simulink model "sim_elicottero"  (R2025b)
settings: Solver=VariableStepAuto  StartTime=0.0  StopTime=200  RelTol=1e-3
values from neighbouring files (symbols this model uses):
  A_nom = double(subs(A_sym_nom, [x;u], [x0;u0]))    [dataset_elicottero.m]
  aero = evalin('base','aero')    [analisi_LQG.m]
  alpha_0 = deg2rad(10)    [dataset_elicottero.m]
  B_ext_nom = [B_nom Bd_nom]    [dataset_elicottero.m]
  beta_0 = 0    [dataset_elicottero.m]
  C_angles = [ ... (first row only)    [actuator_lumped_uncertainty.m]    (also in analisi_montecarlo.m = [1 0 0 0; 0 0 1 0]; dataset_elicottero.m)
  Ddec_phys = [8.48868560985e-05  4.80771131122e-11; -3.04359895869e-06  1.06562367592e-06]    [HINF_controllers.mat]    (also in Hinf_hinfstruct.m = Du *      Ddec_scaled *      Du_inv; Hinf_synthesis_full.m = Du *      Ddec_scaled *      inv(Du))
  den_2nd = [1, 2*zeta*omega_n, omega_n^2]    [dataset_elicottero.m]
  denFalpha = [1 24.6158182311]    [HINF_controllers.mat]
  denFbeta = [1 13.1899797029]    [HINF_controllers.mat]
  F1_0 = u0_nom(1)    [dataset_elicottero.m]
  F2_0 = u0_nom(2)    [dataset_elicottero.m]
  HalphaBeta = (C_angle_meas.'*Vinv*C_angle_meas) \      (C_angle_meas.'*Vinv)    [dataset_elicottero.m]
  K_hinfsyn = minreal(          Du *          K_hinfsyn_scaled *          Dy_inv,          1e-7)    [Hinf_hinfstruct.m]    (also in Hinf_synthesis_full.m = minreal(          Du *          K_hinfsyn_scaled *          )
  K_lqg_2dof = ss(      Ac_ctrl,      Bc_ctrl,      Cc_ctrl,      Dc_ctrl)    [LQG_reg_2DOF.m]
  K_lqg_int = ss(      Ac_ctrl,      [Bcr Bcy],      Cc_ctrl,      Dc_ctrl)    [LQG_con_integratore.m]
  K_mix = minreal(          Du *          K_mix_scaled *          Dy_inv,          1e-7)    [Hinf_hinfstruct.m]    (also in Hinf_synthesis_full.m = minreal(          Du *          K_mix_scaled *          Dy_i)
  K_mu = Du * K_mu_scaled * Dy_inv    [mu_synthesis.m]
  Kalpha_tuned = pid(          alphaScaledToPhys *          Kalpha_tuned_scaled.Kp,          alphaScaledToPhys *          Kalpha_tuned_scaled.Ki,          alphaScaledToPhys *          Kalpha_tuned_scaled.Kd,          Kalpha_tuned_scaled.Tf)    [Hinf_hinfstruct.m]    (also in Hinf_synthesis_full.m = pid(          alphaScaledToPhys * Kalpha_tuned_scaled.Kp,   )
  Kbeta_tuned = pid(          betaScaledToPhys *          Kbeta_tuned_scaled.Kp,          betaScaledToPhys *          Kbeta_tuned_scaled.Ki,          betaScaledToPhys *          Kbeta_tuned_scaled.Kd,          Kbeta_tuned_scaled.Tf)    [Hinf_hinfstruct.m]    (also in Hinf_synthesis_full.m = pid(          betaScaledToPhys * Kbeta_tuned_scaled.Kp,     )
  mx_eq = cos(alpha_0) * cos(beta_0)    [dataset_elicottero.m]
  my_eq = -sin(beta_0)    [dataset_elicottero.m]
  num_2nd = omega_n^2    (= 900)    [dataset_elicottero.m]
  numFalpha = [16.7939294955 590.000844903]    [HINF_controllers.mat]
  numFbeta = [34.4835250476 9.60244651319]    [HINF_controllers.mat]
  P_nom_ext = ss(      A_nom,      B_ext_nom,      Cy,      zeros(3,4))    [dataset_elicottero.m]
  tau_d_nom = 0.02    [dataset_elicottero.m]
  umax = 5    [LQG_con_integratore.m]    (also in LQG_reg_1DOF.m; analisi_montecarlo.m = 2.5; dataset_elicottero.m)
  y_acc_eq = -p.g * sin(alpha_0)    [dataset_elicottero.m]
undefined symbols (not defined in the file or in its folder): act, sensor
libraries: simulink x20, slpidlib x2, cstblocks x2
(part 2 of 2)

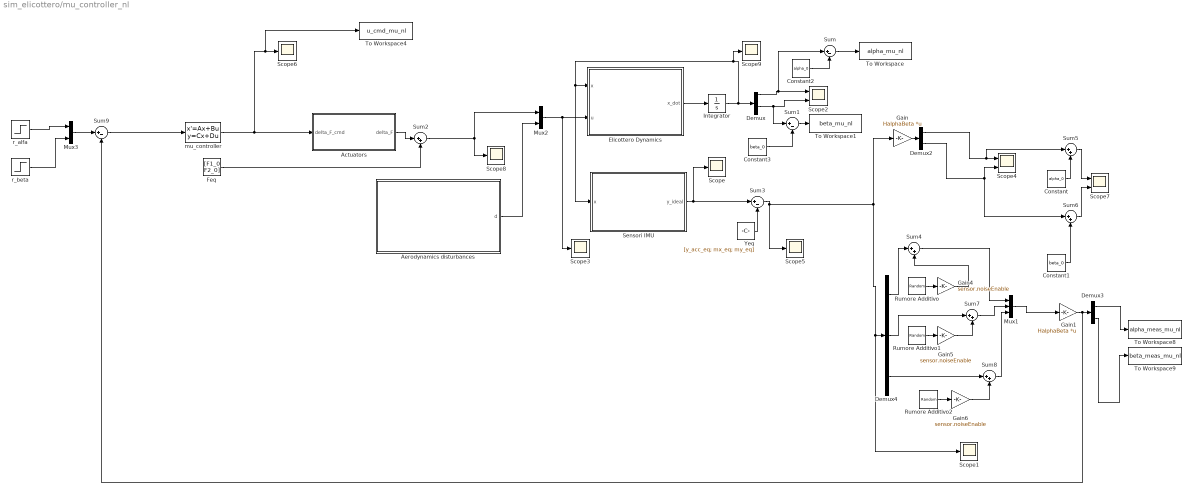
== system sim_elicottero/mu_controller_nl ==
  Actuators : Subsystem
  Aerodynamics disturbances : Subsystem
  Constant : Constant  Value=alpha_0
  Constant1 : Constant  Value=beta_0
  Constant2 : Constant  Value=alpha_0
  Constant3 : Constant  Value=beta_0
  Demux : Demux
  Demux2 : Demux  Outputs=2
  Demux3 : Demux  Outputs=2
  Demux4 : Demux  Outputs=3
  Elicottero Dynamics : MATLAB Function  TreatAsAtomicUnit=on
  Feq : Constant  Value=[F1_0 F2_0]
  Gain : Gain  Gain=HalphaBeta  Multiplication=Matrix(K*u)
  Gain1 : Gain  Gain=HalphaBeta  Multiplication=Matrix(K*u)
  Gain4 : Gain  Gain=sensor.noiseEnable
  Gain5 : Gain  Gain=sensor.noiseEnable
  Gain6 : Gain  Gain=sensor.noiseEnable
  Integrator : Integrator  InitialCondition=[alpha_0; 0; beta_0; 0]
  Mux1 : Mux  Inputs=3
  Mux2 : Mux  Inputs=2
  Mux3 : Mux  Inputs=2
  Rumore Additivo : RandomNumber  Variance=sensor.acc.var  Seed=sensor.seed  SampleTime=sensor.acc.Ts
  Rumore Additivo1 : RandomNumber  Variance=sensor.mag.var  Seed=sensor.seed+1  SampleTime=sensor.mag.Ts
  Rumore Additivo2 : RandomNumber  Variance=sensor.mag.var  Seed=sensor.seed+2  SampleTime=sensor.mag.Ts
  Scope{,1,3,5..6,8..9} (7 alike) : Scope
      Scope settings: ActiveDisplayYMinimum=-2.6695864737629402  ActiveDisplayYMaximum=1.4000873242913907  DataLoggingVariableName=ScopeData14
      Scope1 settings: ActiveDisplayYMinimum=-1.6240661630355766  ActiveDisplayYMaximum=0.25200758348707814  DataLoggingVariableName=ScopeData15
      Scope3 settings: ActiveDisplayYMinimum=-0.066808898460173932  ActiveDisplayYMaximum=0.16260152032849579  DataLoggingVariableName=ScopeData17
      Scope5 settings: ActiveDisplayYMinimum=-0.69850075039123272  ActiveDisplayYMaximum=0.69520204307189137  DataLoggingVariableName=ScopeData20
      Scope6 settings: ActiveDisplayYMinimum=-0.13657354328857155  ActiveDisplayYMaximum=0.3937278655924531  DataLoggingVariableName=ScopeData19
      Scope8 settings: ActiveDisplayYMinimum=-0.16116164249761136  ActiveDisplayYMaximum=0.54820504636646727  DataLoggingVariableName=ScopeData27
      Scope9 settings: ActiveDisplayYMinimum=-0.021816615649929122  ActiveDisplayYMaximum=0.19634954084936207  DataLoggingVariableName=ScopeData28
  Scope2 : Scope  NumInputPorts=2
      settings: ActiveDisplayYMinimum=-0.066338299992033153  ActiveDisplayYMaximum=0.28020406198793696  DataLoggingVariableName=ScopeData16
  Scope4 : Scope  NumInputPorts=2
      settings: ActiveDisplayYMinimum=-0.033068887345671219  ActiveDisplayYMaximum=0.0678695412426075  DataLoggingVariableName=ScopeData18
  Scope7 : Scope  NumInputPorts=2
      settings: ActiveDisplayYMinimum=-0.054885502995600327  ActiveDisplayYMaximum=0.26421908209196954  DataLoggingVariableName=ScopeData26
  Sensori IMU : MATLAB Function  TreatAsAtomicUnit=on
  Sum{,1,3,9} (4 alike) : Sum  Inputs=|+-
  Sum{2,4..8} (6 alike) : Sum  Inputs=|++
  To Workspace : ToWorkspace  VariableName=alpha_mu_nl  SaveFormat=Timeseries  SampleTime=-1
  To Workspace1 : ToWorkspace  VariableName=beta_mu_nl  SaveFormat=Timeseries  SampleTime=-1
  To Workspace4 : ToWorkspace  VariableName=u_cmd_mu_nl  SaveFormat=Timeseries  SampleTime=-1
  To Workspace8 : ToWorkspace  VariableName=alpha_meas_mu_nl  SaveFormat=Timeseries  SampleTime=-1
  To Workspace9 : ToWorkspace  VariableName=beta_meas_mu_nl  SaveFormat=Timeseries  SampleTime=-1
  Yeq : Constant  Value=[y_acc_eq; mx_eq; my_eq]
  mu_controller : StateSpace  A=K_mu.A  B=K_mu.B  C=K_mu.C  D=K_mu.D  InitialCondition=zeros(size(K_mu.A,1),1)
  r_alfa : Step  After=deg2rad(3)  SampleTime=0
  r_beta : Step  After=0  SampleTime=0
  wires:
  mu_controller/1 -> To Workspace4/1, Scope6/1, Actuators/1(delta_F_cmd)
  Mux2/1 -> Scope3/1, Elicottero Dynamics/2(u)
  Aerodynamics disturbances/1(d) -> Mux2/2
  Demux/1 -> Sum/1, Scope2/1
  Demux/3 -> Sum1/1, Scope2/2
  Elicottero Dynamics/1(x_dot) -> Integrator/1
  Integrator/1 -> Scope9/1, Sensori IMU/1(x), Elicottero Dynamics/1(x), Demux/1
  Feq/1 -> Sum2/2
  Sensori IMU/1(y_ideal) -> Sum3/1, Scope/1
  Yeq/1 -> Sum3/2
  Sum7/1 -> Mux1/2
  Constant1/1 -> Sum6/2
  Sum8/1 -> Mux1/3
  Demux4/1 -> Sum4/1
  Rumore Additivo/1 -> Gain4/1
  Gain6/1 -> Sum8/2
  Sum6/1 -> Scope7/2
  Rumore Additivo2/1 -> Gain6/1
  Demux3/2 -> To Workspace9/1
  Rumore Additivo1/1 -> Gain5/1
  Gain5/1 -> Sum7/2
  Demux3/1 -> To Workspace8/1
  Sum4/1 -> Mux1/1
  Demux4/3 -> Sum8/1
  Constant/1 -> Sum5/2
  Demux2/2 -> Sum6/1, Scope4/2
  Demux4/2 -> Sum7/1
  Demux2/1 -> Sum5/1, Scope4/1
  Gain/1 -> Demux2/1
  Sum3/1 -> Demux4/1, Scope1/1, Gain/1, Scope5/1
  Gain4/1 -> Sum4/2
  Sum5/1 -> Scope7/1
  Mux1/1 -> Gain1/1
  Actuators/1(delta_F) -> Sum2/1
  Sum2/1 -> Scope8/1, Mux2/1
  Constant2/1 -> Sum/2
  Sum/1 -> To Workspace/1
  Sum1/1 -> To Workspace1/1
  Constant3/1 -> Sum1/2
  Mux3/1 -> Sum9/1
  r_alfa/1 -> Mux3/1
  r_beta/1 -> Mux3/2
  Sum9/1 -> mu_controller/1
  Gain1/1 -> Sum9/2, Demux3/1

== system sim_elicottero/Hinf_lin/Actuators ==
  delta_F_cmd : Inport
  Band-Limited White Noise : simulink/Sources/Band-Limited White Noise  Cov=act.noisePower_F1  Ts=act.Ts_noise  seed=101
  Band-Limited White Noise1 : simulink/Sources/Band-Limited White Noise  Cov=act.noisePower_F2  Ts=act.Ts_noise  seed=202
  Demux : Demux  Outputs=2
  Gain : Gain  Gain=act.noiseEnable
  Gain1 : Gain  Gain=act.noiseEnable
  Mux : Mux  Inputs=2
  Mux1 : Mux  Inputs=2
  Saturation : Saturate  UpperLimit=act.deltaF1_max  LowerLimit=act.deltaF1_min
  Saturation1 : Saturate  UpperLimit=act.deltaF2_max  LowerLimit=act.deltaF2_min
  Sum1 : Sum  Inputs=|++
  Sum2 : Sum  Inputs=|++
  To Workspace5 : ToWorkspace  VariableName=u_sat_hinf  SaveFormat=Timeseries  SampleTime=-1
  Transfer Fcn : TransferFcn  Numerator=num_2nd  Denominator=den_2nd
  Transfer Fcn1 : TransferFcn  Numerator=num_2nd  Denominator=den_2nd
  Transport Delay1 : TransportDelay  DelayTime=tau_d_nom
  Transport Delay2 : TransportDelay  DelayTime=tau_d_nom
  delta_F : Outport
  wires:
  Gain/1 -> Sum1/2
  Saturation1/1 -> Mux1/2, Transfer Fcn1/1
  Demux/1 -> Saturation/1
  Mux/1 -> delta_F/1
  Transport Delay1/1 -> Sum1/1  "delta_F1"
  Transfer Fcn/1 -> Transport Delay1/1
  Transfer Fcn1/1 -> Transport Delay2/1
  Band-Limited White Noise1/1 -> Gain1/1
  Gain1/1 -> Sum2/2
  Demux/2 -> Saturation1/1
  Transport Delay2/1 -> Sum2/1  "delta_F2"
  delta_F_cmd/1 -> Demux/1
  Band-Limited White Noise/1 -> Gain/1
  Saturation/1 -> Mux1/1, Transfer Fcn/1
  Sum2/1 -> Mux/2
  Sum1/1 -> Mux/1
  Mux1/1 -> To Workspace5/1

== system sim_elicottero/Hinf_lin/Aerodynamics disturbances ==
  Gain : Gain  Gain=aero.enable
  Mux3 : Mux  Inputs=2
  Step : Step  Time=aero.alpha.time  After=aero.alpha.amplitude  SampleTime=0
  Step1 : Step  Time=aero.beta.time  After=aero.beta.amplitude  SampleTime=0
  d : Outport
  wires:
  Step/1 -> Mux3/1
  Mux3/1 -> Gain/1
  Step1/1 -> Mux3/2
  Gain/1 -> d/1

== system sim_elicottero/LQG_1DOF/Actuators ==
  delta_F_cmd : Inport
  Band-Limited White Noise : simulink/Sources/Band-Limited White Noise  Cov=act.noisePower_F1  Ts=act.Ts_noise  seed=101
  Band-Limited White Noise1 : simulink/Sources/Band-Limited White Noise  Cov=act.noisePower_F2  Ts=act.Ts_noise  seed=202
  Demux : Demux  Outputs=2
  Gain : Gain  Gain=act.noiseEnable
  Gain1 : Gain  Gain=act.noiseEnable
  Mux : Mux  Inputs=2
  Mux1 : Mux  Inputs=2
  Saturation : Saturate  UpperLimit=act.deltaF1_max  LowerLimit=act.deltaF1_min
  Saturation1 : Saturate  UpperLimit=act.deltaF2_max  LowerLimit=act.deltaF2_min
  Sum1 : Sum  Inputs=|++
  Sum2 : Sum  Inputs=|++
  To Workspace5 : ToWorkspace  VariableName=u_sat  SaveFormat=Timeseries  SampleTime=-1
  Transfer Fcn : TransferFcn  Numerator=num_2nd  Denominator=den_2nd
  Transfer Fcn1 : TransferFcn  Numerator=num_2nd  Denominator=den_2nd
  Transport Delay1 : TransportDelay  DelayTime=tau_d_nom
  Transport Delay2 : TransportDelay  DelayTime=tau_d_nom
  delta_F : Outport
  wires:
  Gain/1 -> Sum1/2
  Saturation1/1 -> Mux1/2, Transfer Fcn1/1
  Demux/1 -> Saturation/1
  Mux/1 -> delta_F/1
  Transport Delay1/1 -> Sum1/1  "delta_F1"
  Transfer Fcn/1 -> Transport Delay1/1
  Transfer Fcn1/1 -> Transport Delay2/1
  Band-Limited White Noise1/1 -> Gain1/1
  Gain1/1 -> Sum2/2
  Demux/2 -> Saturation1/1
  Transport Delay2/1 -> Sum2/1  "delta_F2"
  delta_F_cmd/1 -> Demux/1
  Band-Limited White Noise/1 -> Gain/1
  Saturation/1 -> Mux1/1, Transfer Fcn/1
  Sum2/1 -> Mux/2
  Sum1/1 -> Mux/1
  Mux1/1 -> To Workspace5/1

== system sim_elicottero/LQG_1DOF/Aerodynamics disturbances ==
  Gain : Gain  Gain=aero.enable
  Mux3 : Mux  Inputs=2
  Step : Step  Time=aero.alpha.time  After=aero.alpha.amplitude  SampleTime=0
  Step1 : Step  Time=aero.beta.time  After=aero.beta.amplitude  SampleTime=0
  d : Outport
  wires:
  Step/1 -> Mux3/1
  Mux3/1 -> Gain/1
  Step1/1 -> Mux3/2
  Gain/1 -> d/1

== system sim_elicottero/LQG_1DOF_nl/Actuators ==
  delta_F_cmd : Inport
  Band-Limited White Noise : simulink/Sources/Band-Limited White Noise  Cov=act.noisePower_F1  Ts=act.Ts_noise  seed=101
  Band-Limited White Noise1 : simulink/Sources/Band-Limited White Noise  Cov=act.noisePower_F2  Ts=act.Ts_noise  seed=202
  Demux : Demux  Outputs=2
  Gain : Gain  Gain=act.noiseEnable
  Gain1 : Gain  Gain=act.noiseEnable
  Mux : Mux  Inputs=2
  Mux1 : Mux  Inputs=2
  Saturation : Saturate  UpperLimit=act.deltaF1_max  LowerLimit=act.deltaF1_min
  Saturation1 : Saturate  UpperLimit=act.deltaF2_max  LowerLimit=act.deltaF2_min
  Sum1 : Sum  Inputs=|++
  Sum2 : Sum  Inputs=|++
  To Workspace5 : ToWorkspace  VariableName=u_sat  SaveFormat=Timeseries  SampleTime=-1
  Transfer Fcn : TransferFcn  Numerator=num_2nd  Denominator=den_2nd
  Transfer Fcn1 : TransferFcn  Numerator=num_2nd  Denominator=den_2nd
  Transport Delay1 : TransportDelay  DelayTime=tau_d_nom
  Transport Delay2 : TransportDelay  DelayTime=tau_d_nom
  delta_F : Outport
  wires:
  Gain/1 -> Sum1/2
  Saturation1/1 -> Mux1/2, Transfer Fcn1/1
  Demux/1 -> Saturation/1
  Mux/1 -> delta_F/1
  Transport Delay1/1 -> Sum1/1  "delta_F1"
  Transfer Fcn/1 -> Transport Delay1/1
  Transfer Fcn1/1 -> Transport Delay2/1
  Band-Limited White Noise1/1 -> Gain1/1
  Gain1/1 -> Sum2/2
  Demux/2 -> Saturation1/1
  Transport Delay2/1 -> Sum2/1  "delta_F2"
  delta_F_cmd/1 -> Demux/1
  Band-Limited White Noise/1 -> Gain/1
  Sum2/1 -> Mux/2
  Sum1/1 -> Mux/1
  Saturation/1 -> Mux1/1, Transfer Fcn/1
  Mux1/1 -> To Workspace5/1

== system sim_elicottero/LQG_1DOF_nl/Aerodynamics disturbances ==
  Gain : Gain  Gain=aero.enable
  Mux3 : Mux  Inputs=2
  Step : Step  Time=aero.alpha.time  After=aero.alpha.amplitude  SampleTime=0
  Step1 : Step  Time=aero.beta.time  After=aero.beta.amplitude  SampleTime=0
  d : Outport
  wires:
  Step/1 -> Mux3/1
  Mux3/1 -> Gain/1
  Step1/1 -> Mux3/2
  Gain/1 -> d/1

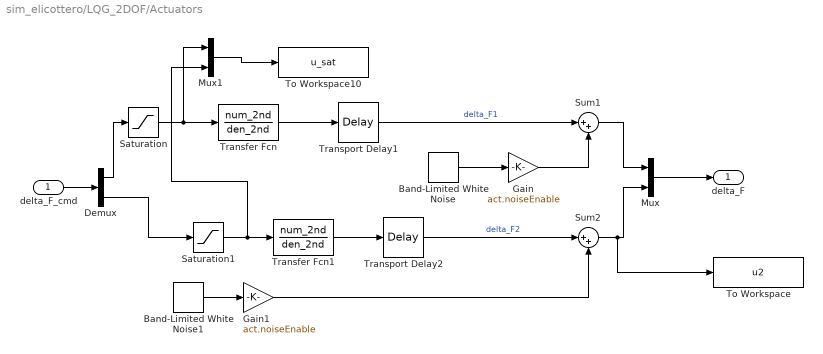
== system sim_elicottero/LQG_2DOF/Actuators ==
  delta_F_cmd : Inport
  Band-Limited White Noise : simulink/Sources/Band-Limited White Noise  Cov=act.noisePower_F1  Ts=act.Ts_noise  seed=101
  Band-Limited White Noise1 : simulink/Sources/Band-Limited White Noise  Cov=act.noisePower_F2  Ts=act.Ts_noise  seed=202
  Demux : Demux  Outputs=2
  Gain : Gain  Gain=act.noiseEnable
  Gain1 : Gain  Gain=act.noiseEnable
  Mux : Mux  Inputs=2
  Mux1 : Mux  Inputs=2
  Saturation : Saturate  UpperLimit=act.deltaF1_max  LowerLimit=act.deltaF1_min
  Saturation1 : Saturate  UpperLimit=act.deltaF2_max  LowerLimit=act.deltaF2_min
  Sum1 : Sum  Inputs=|++
  Sum2 : Sum  Inputs=|++
  To Workspace : ToWorkspace  VariableName=u2  SaveFormat=Timeseries  SampleTime=-1
  To Workspace10 : ToWorkspace  VariableName=u_sat  SaveFormat=Timeseries  SampleTime=-1
  Transfer Fcn : TransferFcn  Numerator=num_2nd  Denominator=den_2nd
  Transfer Fcn1 : TransferFcn  Numerator=num_2nd  Denominator=den_2nd
  Transport Delay1 : TransportDelay  DelayTime=tau_d_nom
  Transport Delay2 : TransportDelay  DelayTime=tau_d_nom
  delta_F : Outport
  wires:
  Gain/1 -> Sum1/2
  Saturation1/1 -> Mux1/2, Transfer Fcn1/1
  Demux/1 -> Saturation/1
  Mux/1 -> delta_F/1
  Transport Delay1/1 -> Sum1/1  "delta_F1"
  Transfer Fcn/1 -> Transport Delay1/1
  Transfer Fcn1/1 -> Transport Delay2/1
  Band-Limited White Noise1/1 -> Gain1/1
  Gain1/1 -> Sum2/2
  Demux/2 -> Saturation1/1
  Transport Delay2/1 -> Sum2/1  "delta_F2"
  delta_F_cmd/1 -> Demux/1
  Band-Limited White Noise/1 -> Gain/1
  Saturation/1 -> Mux1/1, Transfer Fcn/1
  Sum2/1 -> To Workspace/1, Mux/2
  Sum1/1 -> Mux/1
  Mux1/1 -> To Workspace10/1

== system sim_elicottero/LQG_2DOF/Aerodynamics disturbances ==
  Gain : Gain  Gain=aero.enable
  Mux3 : Mux  Inputs=2
  Step : Step  Time=aero.alpha.time  After=aero.alpha.amplitude  SampleTime=0
  Step1 : Step  Time=aero.beta.time  After=aero.beta.amplitude  SampleTime=0
  d : Outport
  wires:
  Step/1 -> Mux3/1
  Mux3/1 -> Gain/1
  Step1/1 -> Mux3/2
  Gain/1 -> d/1

== system sim_elicottero/LQG_2DOF_nl/Actuators ==
  delta_F_cmd : Inport
  Band-Limited White Noise : simulink/Sources/Band-Limited White Noise  Cov=act.noisePower_F1  Ts=act.Ts_noise  seed=101
  Band-Limited White Noise1 : simulink/Sources/Band-Limited White Noise  Cov=act.noisePower_F2  Ts=act.Ts_noise  seed=202
  Demux : Demux  Outputs=2
  Gain : Gain  Gain=act.noiseEnable
  Gain1 : Gain  Gain=act.noiseEnable
  Mux : Mux  Inputs=2
  Saturation : Saturate  UpperLimit=act.deltaF1_max  LowerLimit=act.deltaF1_min
  Saturation1 : Saturate  UpperLimit=act.deltaF2_max  LowerLimit=act.deltaF2_min
  Sum1 : Sum  Inputs=|++
  Sum2 : Sum  Inputs=|++
  To Workspace : ToWorkspace  VariableName=u2  SaveFormat=Timeseries  SampleTime=-1
  Transfer Fcn : TransferFcn  Numerator=num_2nd  Denominator=den_2nd
  Transfer Fcn1 : TransferFcn  Numerator=num_2nd  Denominator=den_2nd
  Transport Delay1 : TransportDelay  DelayTime=tau_d_nom
  Transport Delay2 : TransportDelay  DelayTime=tau_d_nom
  delta_F : Outport
  wires:
  Gain/1 -> Sum1/2
  Saturation1/1 -> Transfer Fcn1/1
  Demux/1 -> Saturation/1
  Mux/1 -> delta_F/1
  Transport Delay1/1 -> Sum1/1  "delta_F1"
  Transfer Fcn/1 -> Transport Delay1/1
  Transfer Fcn1/1 -> Transport Delay2/1
  Band-Limited White Noise1/1 -> Gain1/1
  Gain1/1 -> Sum2/2
  Demux/2 -> Saturation1/1
  Transport Delay2/1 -> Sum2/1  "delta_F2"
  delta_F_cmd/1 -> Demux/1
  Band-Limited White Noise/1 -> Gain/1
  Saturation/1 -> Transfer Fcn/1
  Sum2/1 -> To Workspace/1, Mux/2
  Sum1/1 -> Mux/1

== system sim_elicottero/LQG_2DOF_nl/Aerodynamics disturbances ==
  Gain : Gain  Gain=aero.enable
  Mux3 : Mux  Inputs=2
  Step : Step  Time=aero.alpha.time  After=aero.alpha.amplitude  SampleTime=0
  Step1 : Step  Time=aero.beta.time  After=aero.beta.amplitude  SampleTime=0
  d : Outport
  wires:
  Step/1 -> Mux3/1
  Mux3/1 -> Gain/1
  Step1/1 -> Mux3/2
  Gain/1 -> d/1

== system sim_elicottero/LQG_int/Actuators ==
  delta_F_cmd : Inport
  Band-Limited White Noise : simulink/Sources/Band-Limited White Noise  Cov=act.noisePower_F1  Ts=act.Ts_noise  seed=101
  Band-Limited White Noise1 : simulink/Sources/Band-Limited White Noise  Cov=act.noisePower_F2  Ts=act.Ts_noise  seed=202
  Demux : Demux  Outputs=2
  Gain : Gain  Gain=act.noiseEnable
  Gain1 : Gain  Gain=act.noiseEnable
  Mux : Mux  Inputs=2
  Mux1 : Mux  Inputs=2
  Saturation : Saturate  UpperLimit=act.deltaF1_max  LowerLimit=act.deltaF1_min
  Saturation1 : Saturate  UpperLimit=act.deltaF2_max  LowerLimit=act.deltaF2_min
  Sum1 : Sum  Inputs=|++
  Sum2 : Sum  Inputs=|++
  To Workspace5 : ToWorkspace  VariableName=u_sat  SaveFormat=Timeseries  SampleTime=-1
  Transfer Fcn : TransferFcn  Numerator=num_2nd  Denominator=den_2nd
  Transfer Fcn1 : TransferFcn  Numerator=num_2nd  Denominator=den_2nd
  Transport Delay1 : TransportDelay  DelayTime=tau_d_nom
  Transport Delay2 : TransportDelay  DelayTime=tau_d_nom
  delta_F : Outport
  wires:
  Gain/1 -> Sum1/2
  Saturation1/1 -> Mux1/2, Transfer Fcn1/1
  Demux/1 -> Saturation/1
  Mux/1 -> delta_F/1
  Transport Delay1/1 -> Sum1/1  "delta_F1"
  Transfer Fcn/1 -> Transport Delay1/1
  Transfer Fcn1/1 -> Transport Delay2/1
  Band-Limited White Noise1/1 -> Gain1/1
  Gain1/1 -> Sum2/2
  Demux/2 -> Saturation1/1
  Transport Delay2/1 -> Sum2/1  "delta_F2"
  delta_F_cmd/1 -> Demux/1
  Band-Limited White Noise/1 -> Gain/1
  Saturation/1 -> Mux1/1, Transfer Fcn/1
  Sum2/1 -> Mux/2
  Sum1/1 -> Mux/1
  Mux1/1 -> To Workspace5/1

== system sim_elicottero/LQG_int/Aerodynamics disturbances ==
  Gain : Gain  Gain=aero.enable
  Mux3 : Mux  Inputs=2
  Step : Step  Time=aero.alpha.time  After=aero.alpha.amplitude  SampleTime=0
  Step1 : Step  Time=aero.beta.time  After=aero.beta.amplitude  SampleTime=0
  d : Outport
  wires:
  Step/1 -> Mux3/1
  Mux3/1 -> Gain/1
  Step1/1 -> Mux3/2
  Gain/1 -> d/1

== system sim_elicottero/LQG_int_nl/Actuators ==
  delta_F_cmd : Inport
  Band-Limited White Noise : simulink/Sources/Band-Limited White Noise  Cov=act.noisePower_F1  Ts=act.Ts_noise  seed=101
  Band-Limited White Noise1 : simulink/Sources/Band-Limited White Noise  Cov=act.noisePower_F2  Ts=act.Ts_noise  seed=202
  Demux : Demux  Outputs=2
  Gain : Gain  Gain=act.noiseEnable
  Gain1 : Gain  Gain=act.noiseEnable
  Mux : Mux  Inputs=2
  Mux1 : Mux  Inputs=2
  Saturation : Saturate  UpperLimit=act.deltaF1_max  LowerLimit=act.deltaF1_min
  Saturation1 : Saturate  UpperLimit=act.deltaF2_max  LowerLimit=act.deltaF2_min
  Sum1 : Sum  Inputs=|++
  Sum2 : Sum  Inputs=|++
  To Workspace5 : ToWorkspace  VariableName=u_sat_nl  SaveFormat=Timeseries  SampleTime=-1
  Transfer Fcn : TransferFcn  Numerator=num_2nd  Denominator=den_2nd
  Transfer Fcn1 : TransferFcn  Numerator=num_2nd  Denominator=den_2nd
  Transport Delay1 : TransportDelay  DelayTime=tau_d_nom
  Transport Delay2 : TransportDelay  DelayTime=tau_d_nom
  delta_F : Outport
  wires:
  Gain/1 -> Sum1/2
  Saturation1/1 -> Mux1/2, Transfer Fcn1/1
  Demux/1 -> Saturation/1
  Mux/1 -> delta_F/1
  Transport Delay1/1 -> Sum1/1  "delta_F1"
  Transfer Fcn/1 -> Transport Delay1/1
  Transfer Fcn1/1 -> Transport Delay2/1
  Band-Limited White Noise1/1 -> Gain1/1
  Gain1/1 -> Sum2/2
  Demux/2 -> Saturation1/1
  Transport Delay2/1 -> Sum2/1  "delta_F2"
  delta_F_cmd/1 -> Demux/1
  Band-Limited White Noise/1 -> Gain/1
  Sum2/1 -> Mux/2
  Sum1/1 -> Mux/1
  Saturation/1 -> Mux1/1, Transfer Fcn/1
  Mux1/1 -> To Workspace5/1

== system sim_elicottero/LQG_int_nl/Aerodynamics disturbances ==
  Gain : Gain  Gain=aero.enable
  Mux3 : Mux  Inputs=2
  Step : Step  Time=aero.alpha.time  After=aero.alpha.amplitude  SampleTime=0
  Step1 : Step  Time=aero.beta.time  After=aero.beta.amplitude  SampleTime=0
  d : Outport
  wires:
  Step/1 -> Mux3/1
  Mux3/1 -> Gain/1
  Step1/1 -> Mux3/2
  Gain/1 -> d/1

== system sim_elicottero/mu_controller/Actuators ==
  delta_F_cmd : Inport
  Band-Limited White Noise : simulink/Sources/Band-Limited White Noise  Cov=act.noisePower_F1  Ts=act.Ts_noise  seed=101
  Band-Limited White Noise1 : simulink/Sources/Band-Limited White Noise  Cov=act.noisePower_F2  Ts=act.Ts_noise  seed=202
  Demux : Demux  Outputs=2
  Gain : Gain  Gain=act.noiseEnable
  Gain1 : Gain  Gain=act.noiseEnable
  Mux : Mux  Inputs=2
  Mux1 : Mux  Inputs=2
  Saturation : Saturate  UpperLimit=act.deltaF1_max  LowerLimit=act.deltaF1_min
  Saturation1 : Saturate  UpperLimit=act.deltaF2_max  LowerLimit=act.deltaF2_min
  Sum1 : Sum  Inputs=|++
  Sum2 : Sum  Inputs=|++
  To Workspace5 : ToWorkspace  VariableName=u_sat  SaveFormat=Timeseries  SampleTime=-1
  Transfer Fcn : TransferFcn  Numerator=num_2nd  Denominator=den_2nd
  Transfer Fcn1 : TransferFcn  Numerator=num_2nd  Denominator=den_2nd
  Transport Delay1 : TransportDelay  DelayTime=tau_d_nom
  Transport Delay2 : TransportDelay  DelayTime=tau_d_nom
  delta_F : Outport
  wires:
  Gain/1 -> Sum1/2
  Saturation1/1 -> Mux1/2, Transfer Fcn1/1
  Demux/1 -> Saturation/1
  Mux/1 -> delta_F/1
  Transport Delay1/1 -> Sum1/1  "delta_F1"
  Transfer Fcn/1 -> Transport Delay1/1
  Transfer Fcn1/1 -> Transport Delay2/1
  Band-Limited White Noise1/1 -> Gain1/1
  Gain1/1 -> Sum2/2
  Demux/2 -> Saturation1/1
  Transport Delay2/1 -> Sum2/1  "delta_F2"
  delta_F_cmd/1 -> Demux/1
  Band-Limited White Noise/1 -> Gain/1
  Saturation/1 -> Mux1/1, Transfer Fcn/1
  Sum2/1 -> Mux/2
  Sum1/1 -> Mux/1
  Mux1/1 -> To Workspace5/1

== system sim_elicottero/mu_controller/Aerodynamics disturbances ==
  Gain : Gain  Gain=aero.enable
  Mux3 : Mux  Inputs=2
  Step : Step  Time=aero.alpha.time  After=aero.alpha.amplitude  SampleTime=0
  Step1 : Step  Time=aero.beta.time  After=aero.beta.amplitude  SampleTime=0
  d : Outport
  wires:
  Step/1 -> Mux3/1
  Mux3/1 -> Gain/1
  Step1/1 -> Mux3/2
  Gain/1 -> d/1

== system sim_elicottero/mu_controller_nl/Actuators ==
  delta_F_cmd : Inport
  Band-Limited White Noise : simulink/Sources/Band-Limited White Noise  Cov=act.noisePower_F1  Ts=act.Ts_noise  seed=101
  Band-Limited White Noise1 : simulink/Sources/Band-Limited White Noise  Cov=act.noisePower_F2  Ts=act.Ts_noise  seed=202
  Demux : Demux  Outputs=2
  Gain : Gain  Gain=act.noiseEnable
  Gain1 : Gain  Gain=act.noiseEnable
  Mux : Mux  Inputs=2
  Mux1 : Mux  Inputs=2
  Saturation : Saturate  UpperLimit=act.deltaF1_max  LowerLimit=act.deltaF1_min
  Saturation1 : Saturate  UpperLimit=act.deltaF2_max  LowerLimit=act.deltaF2_min
  Sum1 : Sum  Inputs=|++
  Sum2 : Sum  Inputs=|++
  To Workspace5 : ToWorkspace  VariableName=u_sat_nl  SaveFormat=Timeseries  SampleTime=-1
  Transfer Fcn : TransferFcn  Numerator=num_2nd  Denominator=den_2nd
  Transfer Fcn1 : TransferFcn  Numerator=num_2nd  Denominator=den_2nd
  Transport Delay1 : TransportDelay  DelayTime=tau_d_nom
  Transport Delay2 : TransportDelay  DelayTime=tau_d_nom
  delta_F : Outport
  wires:
  Gain/1 -> Sum1/2
  Saturation1/1 -> Mux1/2, Transfer Fcn1/1
  Demux/1 -> Saturation/1
  Mux/1 -> delta_F/1
  Transport Delay1/1 -> Sum1/1  "delta_F1"
  Transfer Fcn/1 -> Transport Delay1/1
  Transfer Fcn1/1 -> Transport Delay2/1
  Band-Limited White Noise1/1 -> Gain1/1
  Gain1/1 -> Sum2/2
  Demux/2 -> Saturation1/1
  Transport Delay2/1 -> Sum2/1  "delta_F2"
  delta_F_cmd/1 -> Demux/1
  Band-Limited White Noise/1 -> Gain/1
  Sum2/1 -> Mux/2
  Sum1/1 -> Mux/1
  Saturation/1 -> Mux1/1, Transfer Fcn/1
  Mux1/1 -> To Workspace5/1

== system sim_elicottero/mu_controller_nl/Aerodynamics disturbances ==
  Gain : Gain  Gain=aero.enable
  Mux3 : Mux  Inputs=2
  Step : Step  Time=aero.alpha.time  After=aero.alpha.amplitude  SampleTime=0
  Step1 : Step  Time=aero.beta.time  After=aero.beta.amplitude  SampleTime=0
  d : Outport
  wires:
  Step/1 -> Mux3/1
  Mux3/1 -> Gain/1
  Step1/1 -> Mux3/2
  Gain/1 -> d/1

== matlab function sim_elicottero/Hinf_nl/Sensori IMU ==
  data: x input; y_ideal output; p parameter
function y_ideal = sensori_imu(x, p)
    % ESTRAZIONE STATI RILEVANTI
    alpha = x(1);
    beta = x(3);
    
    % EQUAZIONI DEI SENSORI (Misure ideali a 3 uscite)
    y_acc = -p.g * sin(alpha);
    mx = cos(alpha) * cos(beta);
    my = -sin(beta);
    
    % USCITA: Vettore colonna 3x1
    y_ideal = [y_acc; mx; my];
end

== matlab function sim_elicottero/mu_controller_nl/Elicottero Dynamics ==
  data: x input; u input; x_dot output; p parameter
function x_dot = elicottero_dynamics(x, u, p)
    % ESTRAZIONE STATI
    alpha = x(1);
    alpha_dot = x(2);
    beta = x(3);
    beta_dot = x(4);
    
    % ESTRAZIONE INGRESSI

    F1 = u(1);
    F2 = u(2);

    d_alpha = u(3);
    d_beta  = u(4);
                 
    % 1. Vettore velocità angolare nel sistema Body (omega_B)
    % Il Pitch (alpha_dot) ruota attorno all'asse Y_body.
    % Lo Yaw (beta_dot) ruota attorno all'asse Z_inerziale, che proiettato in Body diventa [-sin(alpha); 0; cos(alpha)]
    omega_body = [-beta_dot * sin(alpha); 
                   alpha_dot; 
                   beta_dot * cos(alpha)];
                   
    % 2. Vettore posizione del centro aerodinamico (i rotori a distanza l sull'asse X_body)
    r_cp = [p.l; 0; 0];
    
    % 3. Velocità lineare del corpo dovuta alla rotazione (v = omega x r)
    v_corpo_body = cross(omega_body, r_cp); 
    % (Il risultato analitico sarà: [0; p.l * beta_dot * cos(alpha); -p.l * alpha_dot])
    
    
    % 5. VELOCITÀ RELATIVA VERA (Vento esterno - Velocità del corpo)
    v_rel_body  = - v_corpo_body; 
    v_rel_norm  = norm(v_rel_body);
    
    % Calcolo Forze Aerodinamiche
    % NOTA: Per pulizia del codice, in futuro potresti spostare rho e Cd_A 
    % all'interno della struct dei parametri 'p'
    rho = 1.225; % Densità dell'aria [kg/m^3]
    Cd_A = [0.5; 0.6; 1.2]; % Prodotto Cd * Area per gli assi [X; Y; Z]
    % Bracci da $0.25$ e $0.30$ m: Sono lunghezze tipiche dei bracci di un 
    % elicottero didattico da laboratorio a 2 gradi di libertà, come i 
    % classici modelli Quanser Aero o i TRMS (Twin Rotor MIMO System)
    
    F_drag_body = 0.5 * rho * Cd_A .* v_rel_body * v_rel_norm;
    
    % Calcolo Coppie di Disturbo
    % Assumiamo che la forza aerodinamica agisca con braccio pari a p.l
    tau_wind_alpha = -F_drag_body(3) * p.l; % Forza verticale genera coppia di pitch
    tau_wind_beta  = F_drag_body(2) * p.l; % Forza laterale genera coppia di yaw
    
    % DINAMICA: Inerzia variabile di yaw
    J_beta = p.J_y * sin(alpha)^2 + (p.J_z + p.m*p.l^2)*cos(alpha)^2 + p.I_b;
    
    % EQUAZIONI DEL MOTO (Accelerazioni)
    alpha_ddot = (-p.c_alpha*alpha_dot ...
                  - p.m*p.g*p.l*sin(alpha) ...
                  + p.l*F1*cos(beta) ...
                  + p.eps_p*p.l*F2*sin(beta) ...
                  + d_alpha) / p.J_alpha;

    beta_ddot = (-p.c_beta*beta_dot ...
                 + p.l*F2*cos(alpha) ...
                 + p.eps_y*p.l*F1*sin(alpha) ...
                 + d_beta) / J_beta;
    % USCITA: Vettore colonna delle derivate dello stato
    x_dot = [alpha_dot; alpha_ddot; beta_dot; beta_ddot];
end

== matlab function sim_elicottero/mu_controller_nl/Sensori IMU ==
  data: x input; y_ideal output; p parameter
function y_ideal = sensori_imu(x, p)
    % ESTRAZIONE STATI RILEVANTI
    alpha = x(1);
    beta = x(3);
    
    % EQUAZIONI DEI SENSORI (Misure ideali a 3 uscite)
    y_acc = -p.g * sin(alpha);
    mx = cos(alpha) * cos(beta);
    my = -sin(beta);
    
    % USCITA: Vettore colonna 3x1
    y_ideal = [y_acc; mx; my];
end

== matlab function sim_elicottero/LQG_int_nl/Elicottero Dynamics ==
  data: x input; u input; x_dot output; p parameter
function x_dot = elicottero_dynamics(x, u, p)
    % ESTRAZIONE STATI
    alpha = x(1);
    alpha_dot = x(2);
    beta = x(3);
    beta_dot = x(4);
    
    % ESTRAZIONE INGRESSI

    F1 = u(1);
    F2 = u(2);

    d_alpha = u(3);
    d_beta  = u(4);
                 
    % 1. Vettore velocità angolare nel sistema Body (omega_B)
    % Il Pitch (alpha_dot) ruota attorno all'asse Y_body.
    % Lo Yaw (beta_dot) ruota attorno all'asse Z_inerziale, che proiettato in Body diventa [-sin(alpha); 0; cos(alpha)]
    omega_body = [-beta_dot * sin(alpha); 
                   alpha_dot; 
                   beta_dot * cos(alpha)];
                   
    % 2. Vettore posizione del centro aerodinamico (i rotori a distanza l sull'asse X_body)
    r_cp = [p.l; 0; 0];
    
    % 3. Velocità lineare del corpo dovuta alla rotazione (v = omega x r)
    v_corpo_body = cross(omega_body, r_cp); 
    % (Il risultato analitico sarà: [0; p.l * beta_dot * cos(alpha); -p.l * alpha_dot])
    
    
    % 5. VELOCITÀ RELATIVA VERA (Vento esterno - Velocità del corpo)
    v_rel_body  = - v_corpo_body; 
    v_rel_norm  = norm(v_rel_body);
    
    % Calcolo Forze Aerodinamiche
    % NOTA: Per pulizia del codice, in futuro potresti spostare rho e Cd_A 
    % all'interno della struct dei parametri 'p'
    rho = 1.225; % Densità dell'aria [kg/m^3]
    Cd_A = [0.5; 0.6; 1.2]; % Prodotto Cd * Area per gli assi [X; Y; Z]
    % Bracci da $0.25$ e $0.30$ m: Sono lunghezze tipiche dei bracci di un 
    % elicottero didattico da laboratorio a 2 gradi di libertà, come i 
    % classici modelli Quanser Aero o i TRMS (Twin Rotor MIMO System)
    
    F_drag_body = 0.5 * rho * Cd_A .* v_rel_body * v_rel_norm;
    
    % Calcolo Coppie di Disturbo
    % Assumiamo che la forza aerodinamica agisca con braccio pari a p.l
    tau_wind_alpha = -F_drag_body(3) * p.l; % Forza verticale genera coppia di pitch
    tau_wind_beta  = F_drag_body(2) * p.l; % Forza laterale genera coppia di yaw
    
    % DINAMICA: Inerzia variabile di yaw
    J_beta = p.J_y * sin(alpha)^2 + (p.J_z + p.m*p.l^2)*cos(alpha)^2 + p.I_b;
    
    % EQUAZIONI DEL MOTO (Accelerazioni)
    alpha_ddot = (-p.c_alpha*alpha_dot ...
                  - p.m*p.g*p.l*sin(alpha) ...
                  + p.l*F1*cos(beta) ...
                  + p.eps_p*p.l*F2*sin(beta) ...
                  + d_alpha) / p.J_alpha;

    beta_ddot = (-p.c_beta*beta_dot ...
                 + p.l*F2*cos(alpha) ...
                 + p.eps_y*p.l*F1*sin(alpha) ...
                 + d_beta) / J_beta;
    % USCITA: Vettore colonna delle derivate dello stato
    x_dot = [alpha_dot; alpha_ddot; beta_dot; beta_ddot];
end

== matlab function sim_elicottero/LQG_int_nl/Sensori IMU ==
  data: x input; y_ideal output; p parameter
function y_ideal = sensori_imu(x, p)
    % ESTRAZIONE STATI RILEVANTI
    alpha = x(1);
    beta = x(3);
    
    % EQUAZIONI DEI SENSORI (Misure ideali a 3 uscite)
    y_acc = -p.g * sin(alpha);
    mx = cos(alpha) * cos(beta);
    my = -sin(beta);
    
    % USCITA: Vettore colonna 3x1
    y_ideal = [y_acc; mx; my];
end

== matlab function sim_elicottero/LQG_2DOF_nl/Elicottero Dynamics ==
  data: x input; u input; x_dot output; p parameter
function x_dot = elicottero_dynamics(x, u, p)
    % ESTRAZIONE STATI
    alpha = x(1);
    alpha_dot = x(2);
    beta = x(3);
    beta_dot = x(4);
    
    % ESTRAZIONE INGRESSI

    F1 = u(1);
    F2 = u(2);

    d_alpha = u(3);
    d_beta  = u(4);
                 
    % 1. Vettore velocità angolare nel sistema Body (omega_B)
    % Il Pitch (alpha_dot) ruota attorno all'asse Y_body.
    % Lo Yaw (beta_dot) ruota attorno all'asse Z_inerziale, che proiettato in Body diventa [-sin(alpha); 0; cos(alpha)]
    omega_body = [-beta_dot * sin(alpha); 
                   alpha_dot; 
                   beta_dot * cos(alpha)];
                   
    % 2. Vettore posizione del centro aerodinamico (i rotori a distanza l sull'asse X_body)
    r_cp = [p.l; 0; 0];
    
    % 3. Velocità lineare del corpo dovuta alla rotazione (v = omega x r)
    v_corpo_body = cross(omega_body, r_cp); 
    % (Il risultato analitico sarà: [0; p.l * beta_dot * cos(alpha); -p.l * alpha_dot])
    
    
    % 5. VELOCITÀ RELATIVA VERA (Vento esterno - Velocità del corpo)
    v_rel_body  = - v_corpo_body; 
    v_rel_norm  = norm(v_rel_body);
    
    % Calcolo Forze Aerodinamiche
    % NOTA: Per pulizia del codice, in futuro potresti spostare rho e Cd_A 
    % all'interno della struct dei parametri 'p'
    rho = 1.225; % Densità dell'aria [kg/m^3]
    Cd_A = [0.5; 0.6; 1.2]; % Prodotto Cd * Area per gli assi [X; Y; Z]
    % Bracci da $0.25$ e $0.30$ m: Sono lunghezze tipiche dei bracci di un 
    % elicottero didattico da laboratorio a 2 gradi di libertà, come i 
    % classici modelli Quanser Aero o i TRMS (Twin Rotor MIMO System)
    
    F_drag_body = 0.5 * rho * Cd_A .* v_rel_body * v_rel_norm;
    
    % Calcolo Coppie di Disturbo
    % Assumiamo che la forza aerodinamica agisca con braccio pari a p.l
    tau_wind_alpha = -F_drag_body(3) * p.l; % Forza verticale genera coppia di pitch
    tau_wind_beta  = F_drag_body(2) * p.l; % Forza laterale genera coppia di yaw
    
    % DINAMICA: Inerzia variabile di yaw
    J_beta = p.J_y * sin(alpha)^2 + (p.J_z + p.m*p.l^2)*cos(alpha)^2 + p.I_b;
    
    % EQUAZIONI DEL MOTO (Accelerazioni)
    alpha_ddot = (-p.c_alpha*alpha_dot ...
                  - p.m*p.g*p.l*sin(alpha) ...
                  + p.l*F1*cos(beta) ...
                  + p.eps_p*p.l*F2*sin(beta) ...
                  + d_alpha) / p.J_alpha;

    beta_ddot = (-p.c_beta*beta_dot ...
                 + p.l*F2*cos(alpha) ...
                 + p.eps_y*p.l*F1*sin(alpha) ...
                 + d_beta) / J_beta;
    % USCITA: Vettore colonna delle derivate dello stato
    x_dot = [alpha_dot; alpha_ddot; beta_dot; beta_ddot];
end

== matlab function sim_elicottero/LQG_2DOF_nl/Sensori IMU ==
  data: x input; y_ideal output; p parameter
function y_ideal = sensori_imu(x, p)
    % ESTRAZIONE STATI RILEVANTI
    alpha = x(1);
    beta = x(3);
    
    % EQUAZIONI DEI SENSORI (Misure ideali a 3 uscite)
    y_acc = -p.g * sin(alpha);
    mx = cos(alpha) * cos(beta);
    my = -sin(beta);
    
    % USCITA: Vettore colonna 3x1
    y_ideal = [y_acc; mx; my];
end

== matlab function sim_elicottero/LQG_1DOF_nl/Elicottero Dynamics ==
  data: x input; u input; x_dot output; p parameter
function x_dot = elicottero_dynamics(x, u, p)
    % ESTRAZIONE STATI
    alpha = x(1);
    alpha_dot = x(2);
    beta = x(3);
    beta_dot = x(4);
    
    % ESTRAZIONE INGRESSI

    F1 = u(1);
    F2 = u(2);

    d_alpha = u(3);
    d_beta  = u(4);
                 
    % 1. Vettore velocità angolare nel sistema Body (omega_B)
    % Il Pitch (alpha_dot) ruota attorno all'asse Y_body.
    % Lo Yaw (beta_dot) ruota attorno all'asse Z_inerziale, che proiettato in Body diventa [-sin(alpha); 0; cos(alpha)]
    omega_body = [-beta_dot * sin(alpha); 
                   alpha_dot; 
                   beta_dot * cos(alpha)];
                   
    % 2. Vettore posizione del centro aerodinamico (i rotori a distanza l sull'asse X_body)
    r_cp = [p.l; 0; 0];
    
    % 3. Velocità lineare del corpo dovuta alla rotazione (v = omega x r)
    v_corpo_body = cross(omega_body, r_cp); 
    % (Il risultato analitico sarà: [0; p.l * beta_dot * cos(alpha); -p.l * alpha_dot])
    
    
    % 5. VELOCITÀ RELATIVA VERA (Vento esterno - Velocità del corpo)
    v_rel_body  = - v_corpo_body; 
    v_rel_norm  = norm(v_rel_body);
    
    % Calcolo Forze Aerodinamiche
    % NOTA: Per pulizia del codice, in futuro potresti spostare rho e Cd_A 
    % all'interno della struct dei parametri 'p'
    rho = 1.225; % Densità dell'aria [kg/m^3]
    Cd_A = [0.5; 0.6; 1.2]; % Prodotto Cd * Area per gli assi [X; Y; Z]
    % Bracci da $0.25$ e $0.30$ m: Sono lunghezze tipiche dei bracci di un 
    % elicottero didattico da laboratorio a 2 gradi di libertà, come i 
    % classici modelli Quanser Aero o i TRMS (Twin Rotor MIMO System)
    
    F_drag_body = 0.5 * rho * Cd_A .* v_rel_body * v_rel_norm;
    
    % Calcolo Coppie di Disturbo
    % Assumiamo che la forza aerodinamica agisca con braccio pari a p.l
    tau_wind_alpha = -F_drag_body(3) * p.l; % Forza verticale genera coppia di pitch
    tau_wind_beta  = F_drag_body(2) * p.l; % Forza laterale genera coppia di yaw
    
    % DINAMICA: Inerzia variabile di yaw
    J_beta = p.J_y * sin(alpha)^2 + (p.J_z + p.m*p.l^2)*cos(alpha)^2 + p.I_b;
    
    % EQUAZIONI DEL MOTO (Accelerazioni)
    alpha_ddot = (-p.c_alpha*alpha_dot ...
                  - p.m*p.g*p.l*sin(alpha) ...
                  + p.l*F1*cos(beta) ...
                  + p.eps_p*p.l*F2*sin(beta) ...
                  + d_alpha) / p.J_alpha;

    beta_ddot = (-p.c_beta*beta_dot ...
                 + p.l*F2*cos(alpha) ...
                 + p.eps_y*p.l*F1*sin(alpha) ...
                 + d_beta) / J_beta;
    % USCITA: Vettore colonna delle derivate dello stato
    x_dot = [alpha_dot; alpha_ddot; beta_dot; beta_ddot];
end

== matlab function sim_elicottero/LQG_1DOF_nl/Sensori IMU ==
  data: x input; y_ideal output; p parameter
function y_ideal = sensori_imu(x, p)
    % ESTRAZIONE STATI RILEVANTI
    alpha = x(1);
    beta = x(3);
    
    % EQUAZIONI DEI SENSORI (Misure ideali a 3 uscite)
    y_acc = -p.g * sin(alpha);
    mx = cos(alpha) * cos(beta);
    my = -sin(beta);
    
    % USCITA: Vettore colonna 3x1
    y_ideal = [y_acc; mx; my];
end

== matlab function sim_elicottero/Hinf_nl/Elicottero Dynamics ==
  data: x input; u input; x_dot output; p parameter
function x_dot = elicottero_dynamics(x, u, p)
    % ESTRAZIONE STATI
    alpha = x(1);
    alpha_dot = x(2);
    beta = x(3);
    beta_dot = x(4);
    
    % ESTRAZIONE INGRESSI
    F1 = u(1);
    F2 = u(2);
                 
    % 1. Vettore velocità angolare nel sistema Body (omega_B)
    % Il Pitch (alpha_dot) ruota attorno all'asse Y_body.
    % Lo Yaw (beta_dot) ruota attorno all'asse Z_inerziale, che proiettato in Body diventa [-sin(alpha); 0; cos(alpha)]
    omega_body = [-beta_dot * sin(alpha); 
                   alpha_dot; 
                   beta_dot * cos(alpha)];
                   
    % 2. Vettore posizione del centro aerodinamico (i rotori a distanza l sull'asse X_body)
    r_cp = [p.l; 0; 0];
    
    % 3. Velocità lineare del corpo dovuta alla rotazione (v = omega x r)
    v_corpo_body = cross(omega_body, r_cp); 
    % (Il risultato analitico sarà: [0; p.l * beta_dot * cos(alpha); -p.l * alpha_dot])
    
    
    % 5. VELOCITÀ RELATIVA VERA (Vento esterno - Velocità del corpo)
    v_rel_body  = - v_corpo_body; 
    v_rel_norm  = norm(v_rel_body);
    
    % Calcolo Forze Aerodinamiche
    % NOTA: Per pulizia del codice, in futuro potresti spostare rho e Cd_A 
    % all'interno della struct dei parametri 'p'
    rho = 1.225; % Densità dell'aria [kg/m^3]
    Cd_A = [0.5; 0.6; 1.2]; % Prodotto Cd * Area per gli assi [X; Y; Z]
    % Bracci da $0.25$ e $0.30$ m: Sono lunghezze tipiche dei bracci di un 
    % elicottero didattico da laboratorio a 2 gradi di libertà, come i 
    % classici modelli Quanser Aero o i TRMS (Twin Rotor MIMO System)
    
    F_drag_body = 0.5 * rho * Cd_A .* v_rel_body * v_rel_norm;
    
    % Calcolo Coppie di Disturbo
    % Assumiamo che la forza aerodinamica agisca con braccio pari a p.l
    tau_wind_alpha = -F_drag_body(3) * p.l; % Forza verticale genera coppia di pitch
    tau_wind_beta  = F_drag_body(2) * p.l; % Forza laterale genera coppia di yaw
    
    % DINAMICA: Inerzia variabile di yaw
    J_beta = p.J_y * sin(alpha)^2 + (p.J_z + p.m*p.l^2)*cos(alpha)^2 + p.I_b;
    
    % EQUAZIONI DEL MOTO (Accelerazioni)
    % I momenti del vento sono sommati ai momenti generati dai motori
    alpha_ddot = (-p.c_alpha*alpha_dot - p.m*p.g*p.l*sin(alpha) + p.l*F1*cos(beta) + p.eps_p*p.l*F2*sin(beta) + tau_wind_alpha) / p.J_alpha;
    beta_ddot  = (-p.c_beta*beta_dot + p.l*F2*cos(alpha) + p.eps_y*p.l*F1*sin(alpha) + tau_wind_beta) / J_beta;
    
    
    % USCITA: Vettore colonna delle derivate dello stato
    x_dot = [alpha_dot; alpha_ddot; beta_dot; beta_ddot];
end

== matlab function sim_elicottero/Verifica Dinamica/Elicottero Dynamics ==
  data: x input; u input; x_dot output; p parameter
function x_dot = elicottero_dynamics(x, u, p)
    % ESTRAZIONE STATI
    alpha = x(1);
    alpha_dot = x(2);
    beta = x(3);
    beta_dot = x(4);
    
    % ESTRAZIONE INGRESSI

    F1 = u(1);
    F2 = u(2);

                 
    % 1. Vettore velocità angolare nel sistema Body (omega_B)
    % Il Pitch (alpha_dot) ruota attorno all'asse Y_body.
    % Lo Yaw (beta_dot) ruota attorno all'asse Z_inerziale, che proiettato in Body diventa [-sin(alpha); 0; cos(alpha)]
    omega_body = [-beta_dot * sin(alpha); 
                   alpha_dot; 
                   beta_dot * cos(alpha)];
                   
    % 2. Vettore posizione del centro aerodinamico (i rotori a distanza l sull'asse X_body)
    r_cp = [p.l; 0; 0];
    
    % 3. Velocità lineare del corpo dovuta alla rotazione (v = omega x r)
    v_corpo_body = cross(omega_body, r_cp); 
    % (Il risultato analitico sarà: [0; p.l * beta_dot * cos(alpha); -p.l * alpha_dot])
    
    
    % 5. VELOCITÀ RELATIVA VERA (Vento esterno - Velocità del corpo)
    v_rel_body  = - v_corpo_body; 
    v_rel_norm  = norm(v_rel_body);
    
    % Calcolo Forze Aerodinamiche
    % NOTA: Per pulizia del codice, in futuro potresti spostare rho e Cd_A 
    % all'interno della struct dei parametri 'p'
    rho = 1.225; % Densità dell'aria [kg/m^3]
    Cd_A = [0.5; 0.6; 1.2]; % Prodotto Cd * Area per gli assi [X; Y; Z]
    % Bracci da $0.25$ e $0.30$ m: Sono lunghezze tipiche dei bracci di un 
    % elicottero didattico da laboratorio a 2 gradi di libertà, come i 
    % classici modelli Quanser Aero o i TRMS (Twin Rotor MIMO System)
    
    F_drag_body = 0.5 * rho * Cd_A .* v_rel_body * v_rel_norm;
    
    % Calcolo Coppie di Disturbo
    % Assumiamo che la forza aerodinamica agisca con braccio pari a p.l
    tau_wind_alpha = -F_drag_body(3) * p.l; % Forza verticale genera coppia di pitch
    tau_wind_beta  = F_drag_body(2) * p.l; % Forza laterale genera coppia di yaw
    
    % DINAMICA: Inerzia variabile di yaw
    J_beta = p.J_y * sin(alpha)^2 + (p.J_z + p.m*p.l^2)*cos(alpha)^2 + p.I_b;
    
    % EQUAZIONI DEL MOTO (Accelerazioni)
    alpha_ddot = (-p.c_alpha*alpha_dot ...
                  - p.m*p.g*p.l*sin(alpha) ...
                  + p.l*F1*cos(beta) ...
                  + p.eps_p*p.l*F2*sin(beta) ...
                  ) / p.J_alpha;

    beta_ddot = (-p.c_beta*beta_dot ...
                 + p.l*F2*cos(alpha) ...
                 + p.eps_y*p.l*F1*sin(alpha) ...
                 ) / J_beta;
    % USCITA: Vettore colonna delle derivate dello stato
    x_dot = [alpha_dot; alpha_ddot; beta_dot; beta_ddot];
end
